simulink model "Pedal_Interpretation_exe_gr"  (Simulink 7.0)
settings: Solver=ode4  StartTime=0.0  StopTime=88  FixedStep=0.01  RelTol=1e-3
InitFcn:
  | PedalInterp_para
values from neighbouring files (symbols this model uses):
  ped_min = 5    [PedalInterp_para.m]
  T_max_Brake = 4000    [PedalInterp_para.m]
  TI = 0    [PAS_callback.m]
undefined symbols (not defined in the file or in its folder): fzgbib, m_ab_100pro, m_ab_70pro, PedalInterpretation, v_bereich
libraries: simulink x320
(part 19 of 23)

== system Pedal_Interpretation_exe_gr/Test Specification for PI/SR-PI-02.2 Acceleration pedal interpretation/T_des_Drive does not increase/PAS/none - pass - fail/Arbitration ==
  Pass : Inport  OutDataType=sfix(16)  OutScaling=2^0
  Fail1 : Inport  Port=2  OutDataType=sfix(16)  OutScaling=2^0
  Fail2 : Inport  Port=3  OutDataType=sfix(16)  OutScaling=2^0
  Fail3 : Inport  Port=4  OutDataType=sfix(16)  OutScaling=2^0
  Fail4 : Inport  Port=5  OutDataType=sfix(16)  OutScaling=2^0
  Delay P F1 F3 : Inport  Port=6  OutDataType=sfix(16)  OutScaling=2^0
  Delay F2 : Inport  Port=7  OutDataType=sfix(16)  OutScaling=2^0
  Delay F4 : Inport  Port=8  OutDataType=sfix(16)  OutScaling=2^0
  Max delay : Inport  Port=9  OutDataType=sfix(16)  OutScaling=2^0
  Verdict identification : Subsystem
  Verdict selection : Subsystem
  Verdict : Outport  OutDataType=sfix(16)  OutScaling=2^0
  Delay : Outport  Port=2  OutDataType=sfix(16)  OutScaling=2^0
  wires:
  Pass/1 -> Verdict identification/1(Pass)
  Fail1/1 -> Verdict identification/2(Fail1)
  Fail2/1 -> Verdict identification/3(Fail2)
  Fail3/1 -> Verdict identification/4(Fail3)
  Fail4/1 -> Verdict identification/5(Fail4)
  Delay P F1 F3/1 -> Verdict selection/3(Delay P F1 F3)
  Delay F2/1 -> Verdict selection/4(Delay F2)
  Delay F4/1 -> Verdict selection/5(Delay F4)
  Verdict identification/1(V1) -> Verdict selection/1(V1)
  Verdict identification/2(V2) -> Verdict selection/2(V2)
  Max delay/1 -> Verdict selection/6(Max delay)
  Verdict selection/1(Verdict) -> Verdict/1
  Verdict selection/2(Delay) -> Delay/1

== system Pedal_Interpretation_exe_gr/Test Specification for PI/SR-PI-02.2 Acceleration pedal interpretation/T_des_Drive does not increase/PAS/none - pass - fail/Compute delay ==
  Max Delay : Inport  OutDataType=sfix(16)  OutScaling=2^0
  R AND : Inport  Port=2  OutDataType=sfix(16)  OutScaling=2^0
  Clock : Clock
      settings: Decimation=10
  Clock1 : Clock
      settings: Decimation=10
  Divide : Product  Inputs=/*  OutDataType=sfix(16)  OutScaling=2^-10
  Hold1 : Subsystem  TreatAsAtomicUnit=on
      mask Display: patch(-0.31+[0.4 0.46 0.46 0.54 0.54 0.6 0.6 0.55 0.55 0.45 0.45 0.4],-0.19+[0.85 0.85 0.95 0.95 0.85 0.85 0.87 0.87 0.96 0.96 0.87 0.87],[0 0 0]);
  SimStepSize : Constant  Value=0.01  OutDataType=sfix(16)  OutScaling=2^0
  Subtract : Sum  Inputs=-+  OutDataType=sfix(16)  OutScaling=2^-10
  Subtract1 : Sum  Inputs=+-  OutDataType=sfix(16)  OutScaling=2^-10
  Delay : Outport  OutDataType=sfix(16)  OutScaling=2^0
  wires:
  R AND/1 -> Hold1/1(" ")
  Hold1/1("  ") -> Subtract/2
  Clock1/1 -> Subtract1/1
  Subtract1/1 -> Divide/2
  Subtract/1 -> Subtract1/2
  Clock/1 -> Hold1/2("    ")
  SimStepSize/1 -> Divide/1
  Max Delay/1 -> Subtract/1
  Divide/1 -> Delay/1

== system Pedal_Interpretation_exe_gr/Test Specification for PI/SR-PI-02.2 Acceleration pedal interpretation/T_des_Drive does not increase/PAS/none - pass - fail/Compute delay1 ==
  Max Delay : Inport  OutDataType=sfix(16)  OutScaling=2^0
  R AND/z : Inport  Port=2  OutDataType=sfix(16)  OutScaling=2^0
  Add : Sum  OutDataType=sfix(16)  OutScaling=2^-10
  Clock : Clock
      settings: Decimation=10
  Clock1 : Clock
      settings: Decimation=10
  Divide : Product  Inputs=/*  OutDataType=sfix(16)  OutScaling=2^-10
  Hold1 : Subsystem  TreatAsAtomicUnit=on
      mask Display: patch(-0.31+[0.4 0.46 0.46 0.54 0.54 0.6 0.6 0.55 0.55 0.45 0.45 0.4],-0.19+[0.85 0.85 0.95 0.95 0.85 0.85 0.87 0.87 0.96 0.96 0.87 0.87],[0 0 0]);
  SimStepSize : Constant  Value=0.01  OutDataType=sfix(16)  OutScaling=2^0
  Subtract : Sum  Inputs=-+  OutDataType=sfix(16)  OutScaling=2^-10
  Subtract1 : Sum  Inputs=+-  OutDataType=sfix(16)  OutScaling=2^-10
  Unit : Constant  OutDataType=sfix(16)  OutScaling=2^0
  Delay : Outport  OutDataType=sfix(16)  OutScaling=2^0
  wires:
  Add/1 -> Delay/1
  R AND/z/1 -> Hold1/1(" ")
  Hold1/1("  ") -> Subtract/2
  Clock1/1 -> Subtract1/1
  Subtract1/1 -> Divide/2
  Subtract/1 -> Subtract1/2
  Clock/1 -> Hold1/2("    ")
  SimStepSize/1 -> Divide/1
  Max Delay/1 -> Subtract/1
  Unit/1 -> Add/1
  Divide/1 -> Add/2

== system Pedal_Interpretation_exe_gr/Test Specification for PI/SR-PI-02.2 Acceleration pedal interpretation/T_des_Drive does not increase/PAS/none - pass - fail/Compute delay2 ==
  Max Delay : Inport  OutDataType=sfix(16)  OutScaling=2^0
  Rp & NOT(Ra) : Inport  Port=2  OutDataType=sfix(16)  OutScaling=2^0
  Clock : Clock
      settings: Decimation=10
  Clock1 : Clock
      settings: Decimation=10
  Divide : Product  Inputs=/*  OutDataType=sfix(16)  OutScaling=2^-10
  Hold1 : Subsystem  TreatAsAtomicUnit=on
      mask Display: patch(-0.31+[0.4 0.46 0.46 0.54 0.54 0.6 0.6 0.55 0.55 0.45 0.45 0.4],-0.19+[0.85 0.85 0.95 0.95 0.85 0.85 0.87 0.87 0.96 0.96 0.87 0.87],[0 0 0]);
  SimStepSize : Constant  Value=0.01  OutDataType=sfix(16)  OutScaling=2^0
  Subtract : Sum  Inputs=-+  OutDataType=sfix(16)  OutScaling=2^-10
  Subtract1 : Sum  Inputs=+-  OutDataType=sfix(16)  OutScaling=2^-10
  Delay : Outport  OutDataType=sfix(16)  OutScaling=2^0
  wires:
  Max Delay/1 -> Subtract/1
  SimStepSize/1 -> Divide/1
  Clock/1 -> Hold1/2("    ")
  Subtract/1 -> Subtract1/2
  Subtract1/1 -> Divide/2
  Clock1/1 -> Subtract1/1
  Hold1/1("  ") -> Subtract/2
  Rp & NOT(Ra)/1 -> Hold1/1(" ")
  Divide/1 -> Delay/1

== system Pedal_Interpretation_exe_gr/Test Specification for PI/SR-PI-02.2 Acceleration pedal interpretation/T_des_Drive does not increase/PAS/none - pass - fail/Hold R AND1 ==
  " " : Inport  OutDataType=sfix(16)  OutScaling=2^0
  "    " : Inport  Port=2  OutDataType=sfix(16)  OutScaling=2^0
  Memory : Memory  Orientation=left
  Switch : Switch  Criteria=u2 ~= 0
  "  " : Outport  OutDataType=sfix(16)  OutScaling=2^0
  wires:
  " "/1 -> Switch/2
  "    "/1 -> Switch/1
  Switch/1 -> "  "/1, Memory/1
  Memory/1 -> Switch/3

== system Pedal_Interpretation_exe_gr/Test Specification for PI/SR-PI-02.2 Acceleration pedal interpretation/T_des_Drive does not increase/PAS/none - pass - fail/Hold R AND2 ==
  " " : Inport  OutDataType=sfix(16)  OutScaling=2^0
  "    " : Inport  Port=2  OutDataType=sfix(16)  OutScaling=2^0
  Memory : Memory  Orientation=left
  Switch : Switch  Criteria=u2 ~= 0
  "  " : Outport  OutDataType=sfix(16)  OutScaling=2^0
  wires:
  " "/1 -> Switch/2
  "    "/1 -> Switch/1
  Switch/1 -> "  "/1, Memory/1
  Memory/1 -> Switch/3

== system Pedal_Interpretation_exe_gr/Test Specification for PI/SR-PI-02.2 Acceleration pedal interpretation/T_des_Drive does not increase/PAS/none - pass - fail/Hold R AND3 ==
  " " : Inport  OutDataType=sfix(16)  OutScaling=2^0
  "    " : Inport  Port=2  OutDataType=sfix(16)  OutScaling=2^0
  Memory : Memory  Orientation=left
  Switch : Switch  Criteria=u2 ~= 0
  "  " : Outport  OutDataType=sfix(16)  OutScaling=2^0
  wires:
  Memory/1 -> Switch/3
  Switch/1 -> Memory/1, "  "/1
  "    "/1 -> Switch/1
  " "/1 -> Switch/2

== system Pedal_Interpretation_exe_gr/Test Specification for PI/SR-PI-02.2 Acceleration pedal interpretation/T_des_Drive does not increase/PAS/none - pass - fail/Hold1 ==
  " " : Inport  OutDataType=sfix(16)  OutScaling=2^0
  "    " : Inport  Port=2  OutDataType=sfix(16)  OutScaling=2^0
  Memory : Memory  Orientation=left
  Switch : Switch  Criteria=u2 ~= 0
  "  " : Outport  OutDataType=sfix(16)  OutScaling=2^0
  wires:
  " "/1 -> Switch/2
  "    "/1 -> Switch/1
  Switch/1 -> "  "/1, Memory/1
  Memory/1 -> Switch/3

== system Pedal_Interpretation_exe_gr/Test Specification for PI/SR-PI-02.2 Acceleration pedal interpretation/T_des_Drive does not increase/PAS/none - pass - fail/Hold2 ==
  " " : Inport  OutDataType=sfix(16)  OutScaling=2^0
  "    " : Inport  Port=2  OutDataType=sfix(16)  OutScaling=2^0
  Memory : Memory  Orientation=left
  Switch : Switch  Criteria=u2 ~= 0
  "  " : Outport  OutDataType=sfix(16)  OutScaling=2^0
  wires:
  " "/1 -> Switch/2
  "    "/1 -> Switch/1
  Switch/1 -> "  "/1, Memory/1
  Memory/1 -> Switch/3

== system Pedal_Interpretation_exe_gr/Test Specification for PI/SR-PI-02.2 Acceleration pedal interpretation/T_des_Drive does not increase/PAS/none - pass - fail/Hold3 ==
  " " : Inport  OutDataType=sfix(16)  OutScaling=2^0
  "    " : Inport  Port=2  OutDataType=sfix(16)  OutScaling=2^0
  Memory : Memory  Orientation=left
  Switch : Switch  Criteria=u2 ~= 0
  "  " : Outport  OutDataType=sfix(16)  OutScaling=2^0
  wires:
  Memory/1 -> Switch/3
  Switch/1 -> Memory/1, "  "/1
  "    "/1 -> Switch/1
  " "/1 -> Switch/2

== system Pedal_Interpretation_exe_gr/Test Specification for PI/SR-PI-02.2 Acceleration pedal interpretation/T_des_Drive does not increase/PAS/none - pass - fail/Hold4 ==
  " " : Inport  OutDataType=sfix(16)  OutScaling=2^0
  "    " : Inport  Port=2  OutDataType=sfix(16)  OutScaling=2^0
  Memory : Memory  Orientation=left
  Switch : Switch  Criteria=u2 ~= 0
  "  " : Outport  OutDataType=sfix(16)  OutScaling=2^0
  wires:
  " "/1 -> Switch/2
  "    "/1 -> Switch/1
  Switch/1 -> "  "/1, Memory/1
  Memory/1 -> Switch/3

== system Pedal_Interpretation_exe_gr/Test Specification for PI/SR-PI-02.2 Acceleration pedal interpretation/T_des_Drive does not increase/PAS/none - pass - fail/Hold5 ==
  " " : Inport  OutDataType=sfix(16)  OutScaling=2^0
  "    " : Inport  Port=2  OutDataType=sfix(16)  OutScaling=2^0
  Memory : Memory  Orientation=left
  Switch : Switch  Criteria=u2 ~= 0
  "  " : Outport  OutDataType=sfix(16)  OutScaling=2^0
  wires:
  Memory/1 -> Switch/3
  Switch/1 -> Memory/1, "  "/1
  "    "/1 -> Switch/1
  " "/1 -> Switch/2

== system Pedal_Interpretation_exe_gr/Test Specification for PI/SR-PI-02.2 Acceleration pedal interpretation/T_des_Drive increases/PAS/Delay bus signals/AD delay ==
  In1 : Inport  OutDataType=sfix(16)  OutScaling=2^0
  Delay : Constant  Value=0  OutDataType=sfix(16)  OutScaling=2^0
  Integer Delay : S-Function  FunctionName=sfix_udelay  Parameters=samptime,vinit,NumDelays,1,1,0  mask(Integer Delay){vinit=0.0, samptime=-1, NumDelays=2}
      mask prompts: vinit "Initial condition:"; samptime "Sample time:"; NumDelays "Number of delays:"
      mask help: Delay a signal N sample periods.
      mask init:
      | if isempty(NumDelays)
      |    NumDelays = 1;
      | end
      mask Display: fprintf(' %d\nZ   ',-1*(NumDelays))
  Switch : Switch  Criteria=u2 ~= 0
  Out1 : Outport  OutDataType=sfix(16)  OutScaling=2^0
  wires:
  Integer Delay/1 -> Switch/1
  Delay/1 -> Switch/2
  In1/1 -> Integer Delay/1, Switch/3
  Switch/1 -> Out1/1

== system Pedal_Interpretation_exe_gr/Test Specification for PI/SR-PI-02.2 Acceleration pedal interpretation/T_des_Drive increases/PAS/Delay bus signals/ELL delay ==
  In1 : Inport  OutDataType=sfix(16)  OutScaling=2^0
  Delay : Constant  Value=0  OutDataType=sfix(16)  OutScaling=2^0
  Integer Delay : S-Function  FunctionName=sfix_udelay  Parameters=samptime,vinit,NumDelays,1,1,0  mask(Integer Delay){vinit=0.0, samptime=-1, NumDelays=2}
      mask prompts: vinit "Initial condition:"; samptime "Sample time:"; NumDelays "Number of delays:"
      mask help: Delay a signal N sample periods.
      mask init:
      | if isempty(NumDelays)
      |    NumDelays = 1;
      | end
      mask Display: fprintf(' %d\nZ   ',-1*(NumDelays))
  Switch : Switch  Criteria=u2 ~= 0
  Out1 : Outport  OutDataType=sfix(16)  OutScaling=2^0
  wires:
  Integer Delay/1 -> Switch/1
  Delay/1 -> Switch/2
  In1/1 -> Integer Delay/1, Switch/3
  Switch/1 -> Out1/1

== system Pedal_Interpretation_exe_gr/Test Specification for PI/SR-PI-02.2 Acceleration pedal interpretation/T_des_Drive increases/PAS/Delay bus signals/EUL delay ==
  In1 : Inport  OutDataType=sfix(16)  OutScaling=2^0
  Delay : Constant  Value=0  OutDataType=sfix(16)  OutScaling=2^0
  Integer Delay : S-Function  FunctionName=sfix_udelay  Parameters=samptime,vinit,NumDelays,1,1,0  mask(Integer Delay){vinit=0.0, samptime=-1, NumDelays=2}
      mask prompts: vinit "Initial condition:"; samptime "Sample time:"; NumDelays "Number of delays:"
      mask help: Delay a signal N sample periods.
      mask init:
      | if isempty(NumDelays)
      |    NumDelays = 1;
      | end
      mask Display: fprintf(' %d\nZ   ',-1*(NumDelays))
  Switch : Switch  Criteria=u2 ~= 0
  Out1 : Outport  OutDataType=sfix(16)  OutScaling=2^0
  wires:
  Switch/1 -> Out1/1
  In1/1 -> Switch/3, Integer Delay/1
  Delay/1 -> Switch/2
  Integer Delay/1 -> Switch/1

== system Pedal_Interpretation_exe_gr/Test Specification for PI/SR-PI-02.2 Acceleration pedal interpretation/T_des_Drive increases/PAS/none - pass - fail/Arbitration ==
  Pass : Inport  OutDataType=sfix(16)  OutScaling=2^0
  Fail1 : Inport  Port=2  OutDataType=sfix(16)  OutScaling=2^0
  Fail2 : Inport  Port=3  OutDataType=sfix(16)  OutScaling=2^0
  Fail3 : Inport  Port=4  OutDataType=sfix(16)  OutScaling=2^0
  Fail4 : Inport  Port=5  OutDataType=sfix(16)  OutScaling=2^0
  Delay P F1 F3 : Inport  Port=6  OutDataType=sfix(16)  OutScaling=2^0
  Delay F2 : Inport  Port=7  OutDataType=sfix(16)  OutScaling=2^0
  Delay F4 : Inport  Port=8  OutDataType=sfix(16)  OutScaling=2^0
  Max delay : Inport  Port=9  OutDataType=sfix(16)  OutScaling=2^0
  Verdict identification : Subsystem
  Verdict selection : Subsystem
  Verdict : Outport  OutDataType=sfix(16)  OutScaling=2^0
  Delay : Outport  Port=2  OutDataType=sfix(16)  OutScaling=2^0
  wires:
  Pass/1 -> Verdict identification/1(Pass)
  Fail1/1 -> Verdict identification/2(Fail1)
  Fail2/1 -> Verdict identification/3(Fail2)
  Fail3/1 -> Verdict identification/4(Fail3)
  Fail4/1 -> Verdict identification/5(Fail4)
  Delay P F1 F3/1 -> Verdict selection/3(Delay P F1 F3)
  Delay F2/1 -> Verdict selection/4(Delay F2)
  Delay F4/1 -> Verdict selection/5(Delay F4)
  Verdict identification/1(V1) -> Verdict selection/1(V1)
  Verdict identification/2(V2) -> Verdict selection/2(V2)
  Max delay/1 -> Verdict selection/6(Max delay)
  Verdict selection/1(Verdict) -> Verdict/1
  Verdict selection/2(Delay) -> Delay/1

== system Pedal_Interpretation_exe_gr/Test Specification for PI/SR-PI-02.2 Acceleration pedal interpretation/T_des_Drive increases/PAS/none - pass - fail/Compute delay ==
  Max Delay : Inport  OutDataType=sfix(16)  OutScaling=2^0
  R AND : Inport  Port=2  OutDataType=sfix(16)  OutScaling=2^0
  Clock : Clock
      settings: Decimation=10
  Clock1 : Clock
      settings: Decimation=10
  Divide : Product  Inputs=/*  OutDataType=sfix(16)  OutScaling=2^-10
  Hold1 : Subsystem  TreatAsAtomicUnit=on
      mask Display: patch(-0.31+[0.4 0.46 0.46 0.54 0.54 0.6 0.6 0.55 0.55 0.45 0.45 0.4],-0.19+[0.85 0.85 0.95 0.95 0.85 0.85 0.87 0.87 0.96 0.96 0.87 0.87],[0 0 0]);
  SimStepSize : Constant  Value=0.01  OutDataType=sfix(16)  OutScaling=2^0
  Subtract : Sum  Inputs=-+  OutDataType=sfix(16)  OutScaling=2^-10
  Subtract1 : Sum  Inputs=+-  OutDataType=sfix(16)  OutScaling=2^-10
  Delay : Outport  OutDataType=sfix(16)  OutScaling=2^0
  wires:
  R AND/1 -> Hold1/1(" ")
  Hold1/1("  ") -> Subtract/2
  Clock1/1 -> Subtract1/1
  Subtract1/1 -> Divide/2
  Subtract/1 -> Subtract1/2
  Clock/1 -> Hold1/2("    ")
  SimStepSize/1 -> Divide/1
  Max Delay/1 -> Subtract/1
  Divide/1 -> Delay/1

== system Pedal_Interpretation_exe_gr/Test Specification for PI/SR-PI-02.2 Acceleration pedal interpretation/T_des_Drive increases/PAS/none - pass - fail/Compute delay1 ==
  Max Delay : Inport  OutDataType=sfix(16)  OutScaling=2^0
  R AND/z : Inport  Port=2  OutDataType=sfix(16)  OutScaling=2^0
  Add : Sum  OutDataType=sfix(16)  OutScaling=2^-10
  Clock : Clock
      settings: Decimation=10
  Clock1 : Clock
      settings: Decimation=10
  Divide : Product  Inputs=/*  OutDataType=sfix(16)  OutScaling=2^-10
  Hold1 : Subsystem  TreatAsAtomicUnit=on
      mask Display: patch(-0.31+[0.4 0.46 0.46 0.54 0.54 0.6 0.6 0.55 0.55 0.45 0.45 0.4],-0.19+[0.85 0.85 0.95 0.95 0.85 0.85 0.87 0.87 0.96 0.96 0.87 0.87],[0 0 0]);
  SimStepSize : Constant  Value=0.01  OutDataType=sfix(16)  OutScaling=2^0
  Subtract : Sum  Inputs=-+  OutDataType=sfix(16)  OutScaling=2^-10
  Subtract1 : Sum  Inputs=+-  OutDataType=sfix(16)  OutScaling=2^-10
  Unit : Constant  OutDataType=sfix(16)  OutScaling=2^0
  Delay : Outport  OutDataType=sfix(16)  OutScaling=2^0
  wires:
  Add/1 -> Delay/1
  R AND/z/1 -> Hold1/1(" ")
  Hold1/1("  ") -> Subtract/2
  Clock1/1 -> Subtract1/1
  Subtract1/1 -> Divide/2
  Subtract/1 -> Subtract1/2
  Clock/1 -> Hold1/2("    ")
  SimStepSize/1 -> Divide/1
  Max Delay/1 -> Subtract/1
  Unit/1 -> Add/1
  Divide/1 -> Add/2

== system Pedal_Interpretation_exe_gr/Test Specification for PI/SR-PI-02.2 Acceleration pedal interpretation/T_des_Drive increases/PAS/none - pass - fail/Compute delay2 ==
  Max Delay : Inport  OutDataType=sfix(16)  OutScaling=2^0
  Rp & NOT(Ra) : Inport  Port=2  OutDataType=sfix(16)  OutScaling=2^0
  Clock : Clock
      settings: Decimation=10
  Clock1 : Clock
      settings: Decimation=10
  Divide : Product  Inputs=/*  OutDataType=sfix(16)  OutScaling=2^-10
  Hold1 : Subsystem  TreatAsAtomicUnit=on
      mask Display: patch(-0.31+[0.4 0.46 0.46 0.54 0.54 0.6 0.6 0.55 0.55 0.45 0.45 0.4],-0.19+[0.85 0.85 0.95 0.95 0.85 0.85 0.87 0.87 0.96 0.96 0.87 0.87],[0 0 0]);
  SimStepSize : Constant  Value=0.01  OutDataType=sfix(16)  OutScaling=2^0
  Subtract : Sum  Inputs=-+  OutDataType=sfix(16)  OutScaling=2^-10
  Subtract1 : Sum  Inputs=+-  OutDataType=sfix(16)  OutScaling=2^-10
  Delay : Outport  OutDataType=sfix(16)  OutScaling=2^0
  wires:
  Max Delay/1 -> Subtract/1
  SimStepSize/1 -> Divide/1
  Clock/1 -> Hold1/2("    ")
  Subtract/1 -> Subtract1/2
  Subtract1/1 -> Divide/2
  Clock1/1 -> Subtract1/1
  Hold1/1("  ") -> Subtract/2
  Rp & NOT(Ra)/1 -> Hold1/1(" ")
  Divide/1 -> Delay/1

== system Pedal_Interpretation_exe_gr/Test Specification for PI/SR-PI-02.2 Acceleration pedal interpretation/T_des_Drive increases/PAS/none - pass - fail/Hold R AND1 ==
  " " : Inport  OutDataType=sfix(16)  OutScaling=2^0
  "    " : Inport  Port=2  OutDataType=sfix(16)  OutScaling=2^0
  Memory : Memory  Orientation=left
  Switch : Switch  Criteria=u2 ~= 0
  "  " : Outport  OutDataType=sfix(16)  OutScaling=2^0
  wires:
  " "/1 -> Switch/2
  "    "/1 -> Switch/1
  Switch/1 -> "  "/1, Memory/1
  Memory/1 -> Switch/3

== system Pedal_Interpretation_exe_gr/Test Specification for PI/SR-PI-02.2 Acceleration pedal interpretation/T_des_Drive increases/PAS/none - pass - fail/Hold R AND2 ==
  " " : Inport  OutDataType=sfix(16)  OutScaling=2^0
  "    " : Inport  Port=2  OutDataType=sfix(16)  OutScaling=2^0
  Memory : Memory  Orientation=left
  Switch : Switch  Criteria=u2 ~= 0
  "  " : Outport  OutDataType=sfix(16)  OutScaling=2^0
  wires:
  " "/1 -> Switch/2
  "    "/1 -> Switch/1
  Switch/1 -> "  "/1, Memory/1
  Memory/1 -> Switch/3

== system Pedal_Interpretation_exe_gr/Test Specification for PI/SR-PI-02.2 Acceleration pedal interpretation/T_des_Drive increases/PAS/none - pass - fail/Hold R AND3 ==
  " " : Inport  OutDataType=sfix(16)  OutScaling=2^0
  "    " : Inport  Port=2  OutDataType=sfix(16)  OutScaling=2^0
  Memory : Memory  Orientation=left
  Switch : Switch  Criteria=u2 ~= 0
  "  " : Outport  OutDataType=sfix(16)  OutScaling=2^0
  wires:
  Memory/1 -> Switch/3
  Switch/1 -> Memory/1, "  "/1
  "    "/1 -> Switch/1
  " "/1 -> Switch/2

== system Pedal_Interpretation_exe_gr/Test Specification for PI/SR-PI-02.2 Acceleration pedal interpretation/T_des_Drive increases/PAS/none - pass - fail/Hold1 ==
  " " : Inport  OutDataType=sfix(16)  OutScaling=2^0
  "    " : Inport  Port=2  OutDataType=sfix(16)  OutScaling=2^0
  Memory : Memory  Orientation=left
  Switch : Switch  Criteria=u2 ~= 0
  "  " : Outport  OutDataType=sfix(16)  OutScaling=2^0
  wires:
  " "/1 -> Switch/2
  "    "/1 -> Switch/1
  Switch/1 -> "  "/1, Memory/1
  Memory/1 -> Switch/3

== system Pedal_Interpretation_exe_gr/Test Specification for PI/SR-PI-02.2 Acceleration pedal interpretation/T_des_Drive increases/PAS/none - pass - fail/Hold2 ==
  " " : Inport  OutDataType=sfix(16)  OutScaling=2^0
  "    " : Inport  Port=2  OutDataType=sfix(16)  OutScaling=2^0
  Memory : Memory  Orientation=left
  Switch : Switch  Criteria=u2 ~= 0
  "  " : Outport  OutDataType=sfix(16)  OutScaling=2^0
  wires:
  " "/1 -> Switch/2
  "    "/1 -> Switch/1
  Switch/1 -> "  "/1, Memory/1
  Memory/1 -> Switch/3

== system Pedal_Interpretation_exe_gr/Test Specification for PI/SR-PI-02.2 Acceleration pedal interpretation/T_des_Drive increases/PAS/none - pass - fail/Hold3 ==
  " " : Inport  OutDataType=sfix(16)  OutScaling=2^0
  "    " : Inport  Port=2  OutDataType=sfix(16)  OutScaling=2^0
  Memory : Memory  Orientation=left
  Switch : Switch  Criteria=u2 ~= 0
  "  " : Outport  OutDataType=sfix(16)  OutScaling=2^0
  wires:
  Memory/1 -> Switch/3
  Switch/1 -> Memory/1, "  "/1
  "    "/1 -> Switch/1
  " "/1 -> Switch/2

== system Pedal_Interpretation_exe_gr/Test Specification for PI/SR-PI-02.2 Acceleration pedal interpretation/T_des_Drive increases/PAS/none - pass - fail/Hold4 ==
  " " : Inport  OutDataType=sfix(16)  OutScaling=2^0
  "    " : Inport  Port=2  OutDataType=sfix(16)  OutScaling=2^0
  Memory : Memory  Orientation=left
  Switch : Switch  Criteria=u2 ~= 0
  "  " : Outport  OutDataType=sfix(16)  OutScaling=2^0
  wires:
  " "/1 -> Switch/2
  "    "/1 -> Switch/1
  Switch/1 -> "  "/1, Memory/1
  Memory/1 -> Switch/3

== system Pedal_Interpretation_exe_gr/Test Specification for PI/SR-PI-02.2 Acceleration pedal interpretation/T_des_Drive increases/PAS/none - pass - fail/Hold5 ==
  " " : Inport  OutDataType=sfix(16)  OutScaling=2^0
  "    " : Inport  Port=2  OutDataType=sfix(16)  OutScaling=2^0
  Memory : Memory  Orientation=left
  Switch : Switch  Criteria=u2 ~= 0
  "  " : Outport  OutDataType=sfix(16)  OutScaling=2^0
  wires:
  Memory/1 -> Switch/3
  Switch/1 -> Memory/1, "  "/1
  "    "/1 -> Switch/1
  " "/1 -> Switch/2

== system Pedal_Interpretation_exe_gr/Test Specification for PI/SR-PI-02.2 Acceleration pedal interpretation/T_des_Drive increases /PAS/Delay bus signals/AD delay ==
  In1 : Inport  OutDataType=sfix(16)  OutScaling=2^0
  Delay : Constant  Value=0  OutDataType=sfix(16)  OutScaling=2^0
  Integer Delay : S-Function  FunctionName=sfix_udelay  Parameters=samptime,vinit,NumDelays,1,1,0  mask(Integer Delay){vinit=0.0, samptime=-1, NumDelays=2}
      mask prompts: vinit "Initial condition:"; samptime "Sample time:"; NumDelays "Number of delays:"
      mask help: Delay a signal N sample periods.
      mask init:
      | if isempty(NumDelays)
      |    NumDelays = 1;
      | end
      mask Display: fprintf(' %d\nZ   ',-1*(NumDelays))
  Switch : Switch  Criteria=u2 ~= 0
  Out1 : Outport  OutDataType=sfix(16)  OutScaling=2^0
  wires:
  Integer Delay/1 -> Switch/1
  Delay/1 -> Switch/2
  In1/1 -> Integer Delay/1, Switch/3
  Switch/1 -> Out1/1

== system Pedal_Interpretation_exe_gr/Test Specification for PI/SR-PI-02.2 Acceleration pedal interpretation/T_des_Drive increases /PAS/Delay bus signals/ELL delay ==
  In1 : Inport  OutDataType=sfix(16)  OutScaling=2^0
  Delay : Constant  Value=0  OutDataType=sfix(16)  OutScaling=2^0
  Integer Delay : S-Function  FunctionName=sfix_udelay  Parameters=samptime,vinit,NumDelays,1,1,0  mask(Integer Delay){vinit=0.0, samptime=-1, NumDelays=2}
      mask prompts: vinit "Initial condition:"; samptime "Sample time:"; NumDelays "Number of delays:"
      mask help: Delay a signal N sample periods.
      mask init:
      | if isempty(NumDelays)
      |    NumDelays = 1;
      | end
      mask Display: fprintf(' %d\nZ   ',-1*(NumDelays))
  Switch : Switch  Criteria=u2 ~= 0
  Out1 : Outport  OutDataType=sfix(16)  OutScaling=2^0
  wires:
  Integer Delay/1 -> Switch/1
  Delay/1 -> Switch/2
  In1/1 -> Integer Delay/1, Switch/3
  Switch/1 -> Out1/1

== system Pedal_Interpretation_exe_gr/Test Specification for PI/SR-PI-02.2 Acceleration pedal interpretation/T_des_Drive increases /PAS/Delay bus signals/EUL delay ==
  In1 : Inport  OutDataType=sfix(16)  OutScaling=2^0
  Delay : Constant  Value=0  OutDataType=sfix(16)  OutScaling=2^0
  Integer Delay : S-Function  FunctionName=sfix_udelay  Parameters=samptime,vinit,NumDelays,1,1,0  mask(Integer Delay){vinit=0.0, samptime=-1, NumDelays=2}
      mask prompts: vinit "Initial condition:"; samptime "Sample time:"; NumDelays "Number of delays:"
      mask help: Delay a signal N sample periods.
      mask init:
      | if isempty(NumDelays)
      |    NumDelays = 1;
      | end
      mask Display: fprintf(' %d\nZ   ',-1*(NumDelays))
  Switch : Switch  Criteria=u2 ~= 0
  Out1 : Outport  OutDataType=sfix(16)  OutScaling=2^0
  wires:
  Switch/1 -> Out1/1
  In1/1 -> Switch/3, Integer Delay/1
  Delay/1 -> Switch/2
  Integer Delay/1 -> Switch/1

== system Pedal_Interpretation_exe_gr/Test Specification for PI/SR-PI-02.2 Acceleration pedal interpretation/T_des_Drive increases /PAS/none - pass - fail/Arbitration ==
  Pass : Inport  OutDataType=sfix(16)  OutScaling=2^0
  Fail1 : Inport  Port=2  OutDataType=sfix(16)  OutScaling=2^0
  Fail2 : Inport  Port=3  OutDataType=sfix(16)  OutScaling=2^0
  Fail3 : Inport  Port=4  OutDataType=sfix(16)  OutScaling=2^0
  Fail4 : Inport  Port=5  OutDataType=sfix(16)  OutScaling=2^0
  Delay P F1 F3 : Inport  Port=6  OutDataType=sfix(16)  OutScaling=2^0
  Delay F2 : Inport  Port=7  OutDataType=sfix(16)  OutScaling=2^0
  Delay F4 : Inport  Port=8  OutDataType=sfix(16)  OutScaling=2^0
  Max delay : Inport  Port=9  OutDataType=sfix(16)  OutScaling=2^0
  Verdict identification : Subsystem
  Verdict selection : Subsystem
  Verdict : Outport  OutDataType=sfix(16)  OutScaling=2^0
  Delay : Outport  Port=2  OutDataType=sfix(16)  OutScaling=2^0
  wires:
  Pass/1 -> Verdict identification/1(Pass)
  Fail1/1 -> Verdict identification/2(Fail1)
  Fail2/1 -> Verdict identification/3(Fail2)
  Fail3/1 -> Verdict identification/4(Fail3)
  Fail4/1 -> Verdict identification/5(Fail4)
  Delay P F1 F3/1 -> Verdict selection/3(Delay P F1 F3)
  Delay F2/1 -> Verdict selection/4(Delay F2)
  Delay F4/1 -> Verdict selection/5(Delay F4)
  Verdict identification/1(V1) -> Verdict selection/1(V1)
  Verdict identification/2(V2) -> Verdict selection/2(V2)
  Max delay/1 -> Verdict selection/6(Max delay)
  Verdict selection/1(Verdict) -> Verdict/1
  Verdict selection/2(Delay) -> Delay/1

== system Pedal_Interpretation_exe_gr/Test Specification for PI/SR-PI-02.2 Acceleration pedal interpretation/T_des_Drive increases /PAS/none - pass - fail/Compute delay ==
  Max Delay : Inport  OutDataType=sfix(16)  OutScaling=2^0
  R AND : Inport  Port=2  OutDataType=sfix(16)  OutScaling=2^0
  Clock : Clock
      settings: Decimation=10
  Clock1 : Clock
      settings: Decimation=10
  Divide : Product  Inputs=/*  OutDataType=sfix(16)  OutScaling=2^-10
  Hold1 : Subsystem  TreatAsAtomicUnit=on
      mask Display: patch(-0.31+[0.4 0.46 0.46 0.54 0.54 0.6 0.6 0.55 0.55 0.45 0.45 0.4],-0.19+[0.85 0.85 0.95 0.95 0.85 0.85 0.87 0.87 0.96 0.96 0.87 0.87],[0 0 0]);
  SimStepSize : Constant  Value=0.01  OutDataType=sfix(16)  OutScaling=2^0
  Subtract : Sum  Inputs=-+  OutDataType=sfix(16)  OutScaling=2^-10
  Subtract1 : Sum  Inputs=+-  OutDataType=sfix(16)  OutScaling=2^-10
  Delay : Outport  OutDataType=sfix(16)  OutScaling=2^0
  wires:
  R AND/1 -> Hold1/1(" ")
  Hold1/1("  ") -> Subtract/2
  Clock1/1 -> Subtract1/1
  Subtract1/1 -> Divide/2
  Subtract/1 -> Subtract1/2
  Clock/1 -> Hold1/2("    ")
  SimStepSize/1 -> Divide/1
  Max Delay/1 -> Subtract/1
  Divide/1 -> Delay/1

== system Pedal_Interpretation_exe_gr/Test Specification for PI/SR-PI-02.2 Acceleration pedal interpretation/T_des_Drive increases /PAS/none - pass - fail/Compute delay1 ==
  Max Delay : Inport  OutDataType=sfix(16)  OutScaling=2^0
  R AND/z : Inport  Port=2  OutDataType=sfix(16)  OutScaling=2^0
  Add : Sum  OutDataType=sfix(16)  OutScaling=2^-10
  Clock : Clock
      settings: Decimation=10
  Clock1 : Clock
      settings: Decimation=10
  Divide : Product  Inputs=/*  OutDataType=sfix(16)  OutScaling=2^-10
  Hold1 : Subsystem  TreatAsAtomicUnit=on
      mask Display: patch(-0.31+[0.4 0.46 0.46 0.54 0.54 0.6 0.6 0.55 0.55 0.45 0.45 0.4],-0.19+[0.85 0.85 0.95 0.95 0.85 0.85 0.87 0.87 0.96 0.96 0.87 0.87],[0 0 0]);
  SimStepSize : Constant  Value=0.01  OutDataType=sfix(16)  OutScaling=2^0
  Subtract : Sum  Inputs=-+  OutDataType=sfix(16)  OutScaling=2^-10
  Subtract1 : Sum  Inputs=+-  OutDataType=sfix(16)  OutScaling=2^-10
  Unit : Constant  OutDataType=sfix(16)  OutScaling=2^0
  Delay : Outport  OutDataType=sfix(16)  OutScaling=2^0
  wires:
  Add/1 -> Delay/1
  R AND/z/1 -> Hold1/1(" ")
  Hold1/1("  ") -> Subtract/2
  Clock1/1 -> Subtract1/1
  Subtract1/1 -> Divide/2
  Subtract/1 -> Subtract1/2
  Clock/1 -> Hold1/2("    ")
  SimStepSize/1 -> Divide/1
  Max Delay/1 -> Subtract/1
  Unit/1 -> Add/1
  Divide/1 -> Add/2

== system Pedal_Interpretation_exe_gr/Test Specification for PI/SR-PI-02.2 Acceleration pedal interpretation/T_des_Drive increases /PAS/none - pass - fail/Compute delay2 ==
  Max Delay : Inport  OutDataType=sfix(16)  OutScaling=2^0
  Rp & NOT(Ra) : Inport  Port=2  OutDataType=sfix(16)  OutScaling=2^0
  Clock : Clock
      settings: Decimation=10
  Clock1 : Clock
      settings: Decimation=10
  Divide : Product  Inputs=/*  OutDataType=sfix(16)  OutScaling=2^-10
  Hold1 : Subsystem  TreatAsAtomicUnit=on
      mask Display: patch(-0.31+[0.4 0.46 0.46 0.54 0.54 0.6 0.6 0.55 0.55 0.45 0.45 0.4],-0.19+[0.85 0.85 0.95 0.95 0.85 0.85 0.87 0.87 0.96 0.96 0.87 0.87],[0 0 0]);
  SimStepSize : Constant  Value=0.01  OutDataType=sfix(16)  OutScaling=2^0
  Subtract : Sum  Inputs=-+  OutDataType=sfix(16)  OutScaling=2^-10
  Subtract1 : Sum  Inputs=+-  OutDataType=sfix(16)  OutScaling=2^-10
  Delay : Outport  OutDataType=sfix(16)  OutScaling=2^0
  wires:
  Max Delay/1 -> Subtract/1
  SimStepSize/1 -> Divide/1
  Clock/1 -> Hold1/2("    ")
  Subtract/1 -> Subtract1/2
  Subtract1/1 -> Divide/2
  Clock1/1 -> Subtract1/1
  Hold1/1("  ") -> Subtract/2
  Rp & NOT(Ra)/1 -> Hold1/1(" ")
  Divide/1 -> Delay/1

== system Pedal_Interpretation_exe_gr/Test Specification for PI/SR-PI-02.2 Acceleration pedal interpretation/T_des_Drive increases /PAS/none - pass - fail/Hold R AND1 ==
  " " : Inport  OutDataType=sfix(16)  OutScaling=2^0
  "    " : Inport  Port=2  OutDataType=sfix(16)  OutScaling=2^0
  Memory : Memory  Orientation=left
  Switch : Switch  Criteria=u2 ~= 0
  "  " : Outport  OutDataType=sfix(16)  OutScaling=2^0
  wires:
  " "/1 -> Switch/2
  "    "/1 -> Switch/1
  Switch/1 -> "  "/1, Memory/1
  Memory/1 -> Switch/3

== system Pedal_Interpretation_exe_gr/Test Specification for PI/SR-PI-02.2 Acceleration pedal interpretation/T_des_Drive increases /PAS/none - pass - fail/Hold R AND2 ==
  " " : Inport  OutDataType=sfix(16)  OutScaling=2^0
  "    " : Inport  Port=2  OutDataType=sfix(16)  OutScaling=2^0
  Memory : Memory  Orientation=left
  Switch : Switch  Criteria=u2 ~= 0
  "  " : Outport  OutDataType=sfix(16)  OutScaling=2^0
  wires:
  " "/1 -> Switch/2
  "    "/1 -> Switch/1
  Switch/1 -> "  "/1, Memory/1
  Memory/1 -> Switch/3

== system Pedal_Interpretation_exe_gr/Test Specification for PI/SR-PI-02.2 Acceleration pedal interpretation/T_des_Drive increases /PAS/none - pass - fail/Hold R AND3 ==
  " " : Inport  OutDataType=sfix(16)  OutScaling=2^0
  "    " : Inport  Port=2  OutDataType=sfix(16)  OutScaling=2^0
  Memory : Memory  Orientation=left
  Switch : Switch  Criteria=u2 ~= 0
  "  " : Outport  OutDataType=sfix(16)  OutScaling=2^0
  wires:
  Memory/1 -> Switch/3
  Switch/1 -> Memory/1, "  "/1
  "    "/1 -> Switch/1
  " "/1 -> Switch/2

== system Pedal_Interpretation_exe_gr/Test Specification for PI/SR-PI-02.2 Acceleration pedal interpretation/T_des_Drive increases /PAS/none - pass - fail/Hold1 ==
  " " : Inport  OutDataType=sfix(16)  OutScaling=2^0
  "    " : Inport  Port=2  OutDataType=sfix(16)  OutScaling=2^0
  Memory : Memory  Orientation=left
  Switch : Switch  Criteria=u2 ~= 0
  "  " : Outport  OutDataType=sfix(16)  OutScaling=2^0
  wires:
  " "/1 -> Switch/2
  "    "/1 -> Switch/1
  Switch/1 -> "  "/1, Memory/1
  Memory/1 -> Switch/3

== system Pedal_Interpretation_exe_gr/Test Specification for PI/SR-PI-02.2 Acceleration pedal interpretation/T_des_Drive increases /PAS/none - pass - fail/Hold2 ==
  " " : Inport  OutDataType=sfix(16)  OutScaling=2^0
  "    " : Inport  Port=2  OutDataType=sfix(16)  OutScaling=2^0
  Memory : Memory  Orientation=left
  Switch : Switch  Criteria=u2 ~= 0
  "  " : Outport  OutDataType=sfix(16)  OutScaling=2^0
  wires:
  " "/1 -> Switch/2
  "    "/1 -> Switch/1
  Switch/1 -> "  "/1, Memory/1
  Memory/1 -> Switch/3

== system Pedal_Interpretation_exe_gr/Test Specification for PI/SR-PI-02.2 Acceleration pedal interpretation/T_des_Drive increases /PAS/none - pass - fail/Hold3 ==
  " " : Inport  OutDataType=sfix(16)  OutScaling=2^0
  "    " : Inport  Port=2  OutDataType=sfix(16)  OutScaling=2^0
  Memory : Memory  Orientation=left
  Switch : Switch  Criteria=u2 ~= 0
  "  " : Outport  OutDataType=sfix(16)  OutScaling=2^0
  wires:
  Memory/1 -> Switch/3
  Switch/1 -> Memory/1, "  "/1
  "    "/1 -> Switch/1
  " "/1 -> Switch/2

== system Pedal_Interpretation_exe_gr/Test Specification for PI/SR-PI-02.2 Acceleration pedal interpretation/T_des_Drive increases /PAS/none - pass - fail/Hold4 ==
  " " : Inport  OutDataType=sfix(16)  OutScaling=2^0
  "    " : Inport  Port=2  OutDataType=sfix(16)  OutScaling=2^0
  Memory : Memory  Orientation=left
  Switch : Switch  Criteria=u2 ~= 0
  "  " : Outport  OutDataType=sfix(16)  OutScaling=2^0
  wires:
  " "/1 -> Switch/2
  "    "/1 -> Switch/1
  Switch/1 -> "  "/1, Memory/1
  Memory/1 -> Switch/3

== system Pedal_Interpretation_exe_gr/Test Specification for PI/SR-PI-02.2 Acceleration pedal interpretation/T_des_Drive increases /PAS/none - pass - fail/Hold5 ==
  " " : Inport  OutDataType=sfix(16)  OutScaling=2^0
  "    " : Inport  Port=2  OutDataType=sfix(16)  OutScaling=2^0
  Memory : Memory  Orientation=left
  Switch : Switch  Criteria=u2 ~= 0
  "  " : Outport  OutDataType=sfix(16)  OutScaling=2^0
  wires:
  Memory/1 -> Switch/3
  Switch/1 -> Memory/1, "  "/1
  "    "/1 -> Switch/1
  " "/1 -> Switch/2

== system Pedal_Interpretation_exe_gr/Test Specification for PI/SR-PI-02.2 Acceleration pedal interpretation/v = const & phi_Acc = const/PS/TI/Delays1 ==
  In1 : Inport  OutDataType=sfix(16)  OutScaling=2^0
  Delay : Constant  Value=0  OutDataType=sfix(16)  OutScaling=2^0
  Integer Delay : S-Function  FunctionName=sfix_udelay  Parameters=samptime,vinit,NumDelays,1,1,0  mask(Integer Delay){vinit=0.0, samptime=-1, NumDelays=15}
      mask prompts: vinit "Initial condition:"; samptime "Sample time:"; NumDelays "Number of delays:"
      mask help: Delay a signal N sample periods.
      mask init:
      | if isempty(NumDelays)
      |    NumDelays = 1;
      | end
      mask Display: fprintf(' %d\nZ   ',-1*(NumDelays))
  Switch : Switch  Criteria=u2 ~= 0
  Out1 : Outport  OutDataType=sfix(16)  OutScaling=2^0
  wires:
  Integer Delay/1 -> Switch/1
  Delay/1 -> Switch/2
  In1/1 -> Integer Delay/1, Switch/3
  Switch/1 -> Out1/1

== system Pedal_Interpretation_exe_gr/Test Specification for PI/SR-PI-02.2 Acceleration pedal interpretation/v = const & phi_Acc = const/PS/TI/Delays2 ==
  In1 : Inport  OutDataType=sfix(16)  OutScaling=2^0
  Delay : Constant  Value=0  OutDataType=sfix(16)  OutScaling=2^0
  Integer Delay : S-Function  FunctionName=sfix_udelay  Parameters=samptime,vinit,NumDelays,1,1,0  mask(Integer Delay){vinit=0.0, samptime=-1, NumDelays=15}
      mask prompts: vinit "Initial condition:"; samptime "Sample time:"; NumDelays "Number of delays:"
      mask help: Delay a signal N sample periods.
      mask init:
      | if isempty(NumDelays)
      |    NumDelays = 1;
      | end
      mask Display: fprintf(' %d\nZ   ',-1*(NumDelays))
  Switch : Switch  Criteria=u2 ~= 0
  Out1 : Outport  OutDataType=sfix(16)  OutScaling=2^0
  wires:
  Integer Delay/1 -> Switch/1
  Delay/1 -> Switch/2
  In1/1 -> Integer Delay/1, Switch/3
  Switch/1 -> Out1/1

== system Pedal_Interpretation_exe_gr/Test Specification for PI/SR-PI-02.2 Acceleration pedal interpretation/v = const & phi_Acc = const/PS/TID/Hold ==
  " " : Inport  OutDataType=sfix(16)  OutScaling=2^0
  "    " : Inport  Port=2  OutDataType=sfix(16)  OutScaling=2^0
  Memory : Memory  Orientation=left
  Switch : Switch  Criteria=u2 ~= 0
  "  " : Outport  OutDataType=sfix(16)  OutScaling=2^0
  wires:
  " "/1 -> Switch/2
  "    "/1 -> Switch/1
  Switch/1 -> "  "/1, Memory/1
  Memory/1 -> Switch/3

== system Pedal_Interpretation_exe_gr/Test Specification for PI/SR-PI-02.2 Acceleration pedal interpretation/v = const & phi_Acc decreases & T_des_Drive < 0/PS/TI/Delays1 ==
  In1 : Inport  OutDataType=sfix(16)  OutScaling=2^0
  Delay : Constant  Value=0  OutDataType=sfix(16)  OutScaling=2^0
  Integer Delay : S-Function  FunctionName=sfix_udelay  Parameters=samptime,vinit,NumDelays,1,1,0  mask(Integer Delay){vinit=0.0, samptime=-1, NumDelays=15}
      mask prompts: vinit "Initial condition:"; samptime "Sample time:"; NumDelays "Number of delays:"
      mask help: Delay a signal N sample periods.
      mask init:
      | if isempty(NumDelays)
      |    NumDelays = 1;
      | end
      mask Display: fprintf(' %d\nZ   ',-1*(NumDelays))
  Switch : Switch  Criteria=u2 ~= 0
  Out1 : Outport  OutDataType=sfix(16)  OutScaling=2^0
  wires:
  Integer Delay/1 -> Switch/1
  Delay/1 -> Switch/2
  In1/1 -> Integer Delay/1, Switch/3
  Switch/1 -> Out1/1

== system Pedal_Interpretation_exe_gr/Test Specification for PI/SR-PI-02.2 Acceleration pedal interpretation/v = const & phi_Acc decreases & T_des_Drive < 0/PS/TI/Delays2 ==
  In1 : Inport  OutDataType=sfix(16)  OutScaling=2^0
  Delay : Constant  Value=0  OutDataType=sfix(16)  OutScaling=2^0
  Integer Delay : S-Function  FunctionName=sfix_udelay  Parameters=samptime,vinit,NumDelays,1,1,0  mask(Integer Delay){vinit=0.0, samptime=-1, NumDelays=15}
      mask prompts: vinit "Initial condition:"; samptime "Sample time:"; NumDelays "Number of delays:"
      mask help: Delay a signal N sample periods.
      mask init:
      | if isempty(NumDelays)
      |    NumDelays = 1;
      | end
      mask Display: fprintf(' %d\nZ   ',-1*(NumDelays))
  Switch : Switch  Criteria=u2 ~= 0
  Out1 : Outport  OutDataType=sfix(16)  OutScaling=2^0
  wires:
  Integer Delay/1 -> Switch/1
  Delay/1 -> Switch/2
  In1/1 -> Integer Delay/1, Switch/3
  Switch/1 -> Out1/1

== system Pedal_Interpretation_exe_gr/Test Specification for PI/SR-PI-02.2 Acceleration pedal interpretation/v = const & phi_Acc decreases & T_des_Drive < 0/PS/TI/Delays3 ==
  In1 : Inport  OutDataType=sfix(16)  OutScaling=2^0
  Delay : Constant  Value=0  OutDataType=sfix(16)  OutScaling=2^0
  Integer Delay : S-Function  FunctionName=sfix_udelay  Parameters=samptime,vinit,NumDelays,1,1,0  mask(Integer Delay){vinit=0.0, samptime=-1, NumDelays=2}
      mask prompts: vinit "Initial condition:"; samptime "Sample time:"; NumDelays "Number of delays:"
      mask help: Delay a signal N sample periods.
      mask init:
      | if isempty(NumDelays)
      |    NumDelays = 1;
      | end
      mask Display: fprintf(' %d\nZ   ',-1*(NumDelays))
  Switch : Switch  Criteria=u2 ~= 0
  Out1 : Outport  OutDataType=sfix(16)  OutScaling=2^0
  wires:
  Integer Delay/1 -> Switch/1
  Delay/1 -> Switch/2
  In1/1 -> Integer Delay/1, Switch/3
  Switch/1 -> Out1/1

== system Pedal_Interpretation_exe_gr/Test Specification for PI/SR-PI-02.2 Acceleration pedal interpretation/v = const & phi_Acc decreases & T_des_Drive < 0/PS/TID/Hold ==
  " " : Inport  OutDataType=sfix(16)  OutScaling=2^0
  "    " : Inport  Port=2  OutDataType=sfix(16)  OutScaling=2^0
  Memory : Memory  Orientation=left
  Switch : Switch  Criteria=u2 ~= 0
  "  " : Outport  OutDataType=sfix(16)  OutScaling=2^0
  wires:
  " "/1 -> Switch/2
  "    "/1 -> Switch/1
  Switch/1 -> "  "/1, Memory/1
  Memory/1 -> Switch/3

== system Pedal_Interpretation_exe_gr/Test Specification for PI/SR-PI-02.2 Acceleration pedal interpretation/v = const & phi_Acc decreases & T_des_Drive >= 0/PS/TI/Delays1 ==
  In1 : Inport  OutDataType=sfix(16)  OutScaling=2^0
  Delay : Constant  Value=0  OutDataType=sfix(16)  OutScaling=2^0
  Integer Delay : S-Function  FunctionName=sfix_udelay  Parameters=samptime,vinit,NumDelays,1,1,0  mask(Integer Delay){vinit=0.0, samptime=-1, NumDelays=15}
      mask prompts: vinit "Initial condition:"; samptime "Sample time:"; NumDelays "Number of delays:"
      mask help: Delay a signal N sample periods.
      mask init:
      | if isempty(NumDelays)
      |    NumDelays = 1;
      | end
      mask Display: fprintf(' %d\nZ   ',-1*(NumDelays))
  Switch : Switch  Criteria=u2 ~= 0
  Out1 : Outport  OutDataType=sfix(16)  OutScaling=2^0
  wires:
  Integer Delay/1 -> Switch/1
  Delay/1 -> Switch/2
  In1/1 -> Integer Delay/1, Switch/3
  Switch/1 -> Out1/1

== system Pedal_Interpretation_exe_gr/Test Specification for PI/SR-PI-02.2 Acceleration pedal interpretation/v = const & phi_Acc decreases & T_des_Drive >= 0/PS/TI/Delays2 ==
  In1 : Inport  OutDataType=sfix(16)  OutScaling=2^0
  Delay : Constant  Value=0  OutDataType=sfix(16)  OutScaling=2^0
  Integer Delay : S-Function  FunctionName=sfix_udelay  Parameters=samptime,vinit,NumDelays,1,1,0  mask(Integer Delay){vinit=0.0, samptime=-1, NumDelays=15}
      mask prompts: vinit "Initial condition:"; samptime "Sample time:"; NumDelays "Number of delays:"
      mask help: Delay a signal N sample periods.
      mask init:
      | if isempty(NumDelays)
      |    NumDelays = 1;
      | end
      mask Display: fprintf(' %d\nZ   ',-1*(NumDelays))
  Switch : Switch  Criteria=u2 ~= 0
  Out1 : Outport  OutDataType=sfix(16)  OutScaling=2^0
  wires:
  Integer Delay/1 -> Switch/1
  Delay/1 -> Switch/2
  In1/1 -> Integer Delay/1, Switch/3
  Switch/1 -> Out1/1

== system Pedal_Interpretation_exe_gr/Test Specification for PI/SR-PI-02.2 Acceleration pedal interpretation/v = const & phi_Acc decreases & T_des_Drive >= 0/PS/TI/Delays3 ==
  In1 : Inport  OutDataType=sfix(16)  OutScaling=2^0
  Delay : Constant  Value=0  OutDataType=sfix(16)  OutScaling=2^0
  Integer Delay : S-Function  FunctionName=sfix_udelay  Parameters=samptime,vinit,NumDelays,1,1,0  mask(Integer Delay){vinit=0.0, samptime=-1, NumDelays=2}
      mask prompts: vinit "Initial condition:"; samptime "Sample time:"; NumDelays "Number of delays:"
      mask help: Delay a signal N sample periods.
      mask init:
      | if isempty(NumDelays)
      |    NumDelays = 1;
      | end
      mask Display: fprintf(' %d\nZ   ',-1*(NumDelays))
  Switch : Switch  Criteria=u2 ~= 0
  Out1 : Outport  OutDataType=sfix(16)  OutScaling=2^0
  wires:
  Integer Delay/1 -> Switch/1
  Delay/1 -> Switch/2
  In1/1 -> Integer Delay/1, Switch/3
  Switch/1 -> Out1/1

== system Pedal_Interpretation_exe_gr/Test Specification for PI/SR-PI-02.2 Acceleration pedal interpretation/v = const & phi_Acc decreases & T_des_Drive >= 0/PS/TID/Hold ==
  " " : Inport  OutDataType=sfix(16)  OutScaling=2^0
  "    " : Inport  Port=2  OutDataType=sfix(16)  OutScaling=2^0
  Memory : Memory  Orientation=left
  Switch : Switch  Criteria=u2 ~= 0
  "  " : Outport  OutDataType=sfix(16)  OutScaling=2^0
  wires:
  " "/1 -> Switch/2
  "    "/1 -> Switch/1
  Switch/1 -> "  "/1, Memory/1
  Memory/1 -> Switch/3

== system Pedal_Interpretation_exe_gr/Test Specification for PI/SR-PI-02.2 Acceleration pedal interpretation/v = const & phi_Acc increases & T_des_Drive < 0/PS/TI/Delays1 ==
  In1 : Inport  OutDataType=sfix(16)  OutScaling=2^0
  Delay : Constant  Value=0  OutDataType=sfix(16)  OutScaling=2^0
  Integer Delay : S-Function  FunctionName=sfix_udelay  Parameters=samptime,vinit,NumDelays,1,1,0  mask(Integer Delay){vinit=0.0, samptime=-1, NumDelays=15}
      mask prompts: vinit "Initial condition:"; samptime "Sample time:"; NumDelays "Number of delays:"
      mask help: Delay a signal N sample periods.
      mask init:
      | if isempty(NumDelays)
      |    NumDelays = 1;
      | end
      mask Display: fprintf(' %d\nZ   ',-1*(NumDelays))
  Switch : Switch  Criteria=u2 ~= 0
  Out1 : Outport  OutDataType=sfix(16)  OutScaling=2^0
  wires:
  Integer Delay/1 -> Switch/1
  Delay/1 -> Switch/2
  In1/1 -> Integer Delay/1, Switch/3
  Switch/1 -> Out1/1

== system Pedal_Interpretation_exe_gr/Test Specification for PI/SR-PI-02.2 Acceleration pedal interpretation/v = const & phi_Acc increases & T_des_Drive < 0/PS/TI/Delays2 ==
  In1 : Inport  OutDataType=sfix(16)  OutScaling=2^0
  Delay : Constant  Value=0  OutDataType=sfix(16)  OutScaling=2^0
  Integer Delay : S-Function  FunctionName=sfix_udelay  Parameters=samptime,vinit,NumDelays,1,1,0  mask(Integer Delay){vinit=0.0, samptime=-1, NumDelays=15}
      mask prompts: vinit "Initial condition:"; samptime "Sample time:"; NumDelays "Number of delays:"
      mask help: Delay a signal N sample periods.
      mask init:
      | if isempty(NumDelays)
      |    NumDelays = 1;
      | end
      mask Display: fprintf(' %d\nZ   ',-1*(NumDelays))
  Switch : Switch  Criteria=u2 ~= 0
  Out1 : Outport  OutDataType=sfix(16)  OutScaling=2^0
  wires:
  Integer Delay/1 -> Switch/1
  Delay/1 -> Switch/2
  In1/1 -> Integer Delay/1, Switch/3
  Switch/1 -> Out1/1

== system Pedal_Interpretation_exe_gr/Test Specification for PI/SR-PI-02.2 Acceleration pedal interpretation/v = const & phi_Acc increases & T_des_Drive < 0/PS/TI/Delays3 ==
  In1 : Inport  OutDataType=sfix(16)  OutScaling=2^0
  Delay : Constant  Value=2  OutDataType=sfix(16)  OutScaling=2^0
  Integer Delay : S-Function  FunctionName=sfix_udelay  Parameters=samptime,vinit,NumDelays,1,1,0  mask(Integer Delay){vinit=0.0, samptime=-1, NumDelays=2}
      mask prompts: vinit "Initial condition:"; samptime "Sample time:"; NumDelays "Number of delays:"
      mask help: Delay a signal N sample periods.
      mask init:
      | if isempty(NumDelays)
      |    NumDelays = 1;
      | end
      mask Display: fprintf(' %d\nZ   ',-1*(NumDelays))
  Switch : Switch  Criteria=u2 ~= 0
  Out1 : Outport  OutDataType=sfix(16)  OutScaling=2^0
  wires:
  Integer Delay/1 -> Switch/1
  Delay/1 -> Switch/2
  In1/1 -> Integer Delay/1, Switch/3
  Switch/1 -> Out1/1

== system Pedal_Interpretation_exe_gr/Test Specification for PI/SR-PI-02.2 Acceleration pedal interpretation/v = const & phi_Acc increases & T_des_Drive < 0/PS/TID/Hold ==
  " " : Inport  OutDataType=sfix(16)  OutScaling=2^0
  "    " : Inport  Port=2  OutDataType=sfix(16)  OutScaling=2^0
  Memory : Memory  Orientation=left
  Switch : Switch  Criteria=u2 ~= 0
  "  " : Outport  OutDataType=sfix(16)  OutScaling=2^0
  wires:
  " "/1 -> Switch/2
  "    "/1 -> Switch/1
  Switch/1 -> "  "/1, Memory/1
  Memory/1 -> Switch/3

== system Pedal_Interpretation_exe_gr/Test Specification for PI/SR-PI-02.2 Acceleration pedal interpretation/v = const & phi_Acc increases & T_des_Drive >= 0/PS/TI/Delays1 ==
  In1 : Inport  OutDataType=sfix(16)  OutScaling=2^0
  Delay : Constant  Value=0  OutDataType=sfix(16)  OutScaling=2^0
  Integer Delay : S-Function  FunctionName=sfix_udelay  Parameters=samptime,vinit,NumDelays,1,1,0  mask(Integer Delay){vinit=0.0, samptime=-1, NumDelays=15}
      mask prompts: vinit "Initial condition:"; samptime "Sample time:"; NumDelays "Number of delays:"
      mask help: Delay a signal N sample periods.
      mask init:
      | if isempty(NumDelays)
      |    NumDelays = 1;
      | end
      mask Display: fprintf(' %d\nZ   ',-1*(NumDelays))
  Switch : Switch  Criteria=u2 ~= 0
  Out1 : Outport  OutDataType=sfix(16)  OutScaling=2^0
  wires:
  Integer Delay/1 -> Switch/1
  Delay/1 -> Switch/2
  In1/1 -> Integer Delay/1, Switch/3
  Switch/1 -> Out1/1

== system Pedal_Interpretation_exe_gr/Test Specification for PI/SR-PI-02.2 Acceleration pedal interpretation/v = const & phi_Acc increases & T_des_Drive >= 0/PS/TI/Delays2 ==
  In1 : Inport  OutDataType=sfix(16)  OutScaling=2^0
  Delay : Constant  Value=0  OutDataType=sfix(16)  OutScaling=2^0
  Integer Delay : S-Function  FunctionName=sfix_udelay  Parameters=samptime,vinit,NumDelays,1,1,0  mask(Integer Delay){vinit=0.0, samptime=-1, NumDelays=15}
      mask prompts: vinit "Initial condition:"; samptime "Sample time:"; NumDelays "Number of delays:"
      mask help: Delay a signal N sample periods.
      mask init:
      | if isempty(NumDelays)
      |    NumDelays = 1;
      | end
      mask Display: fprintf(' %d\nZ   ',-1*(NumDelays))
  Switch : Switch  Criteria=u2 ~= 0
  Out1 : Outport  OutDataType=sfix(16)  OutScaling=2^0
  wires:
  Integer Delay/1 -> Switch/1
  Delay/1 -> Switch/2
  In1/1 -> Integer Delay/1, Switch/3
  Switch/1 -> Out1/1

== system Pedal_Interpretation_exe_gr/Test Specification for PI/SR-PI-02.2 Acceleration pedal interpretation/v = const & phi_Acc increases & T_des_Drive >= 0/PS/TI/Delays3 ==
  In1 : Inport  OutDataType=sfix(16)  OutScaling=2^0
  Delay : Constant  Value=2  OutDataType=sfix(16)  OutScaling=2^0
  Integer Delay : S-Function  FunctionName=sfix_udelay  Parameters=samptime,vinit,NumDelays,1,1,0  mask(Integer Delay){vinit=0.0, samptime=-1, NumDelays=2}
      mask prompts: vinit "Initial condition:"; samptime "Sample time:"; NumDelays "Number of delays:"
      mask help: Delay a signal N sample periods.
      mask init:
      | if isempty(NumDelays)
      |    NumDelays = 1;
      | end
      mask Display: fprintf(' %d\nZ   ',-1*(NumDelays))
  Switch : Switch  Criteria=u2 ~= 0
  Out1 : Outport  OutDataType=sfix(16)  OutScaling=2^0
  wires:
  Integer Delay/1 -> Switch/1
  Delay/1 -> Switch/2
  In1/1 -> Integer Delay/1, Switch/3
  Switch/1 -> Out1/1
